simulink model "ControlModel"  (R2020b)
settings: Solver=VariableStepAuto  StartTime=0.0  StopTime=3  FixedStep=0.00001  RelTol=1e-3
InitFcn:
  | s = tf('s');
  | Telec = 1/10000000;
  | Tmech = Telec * 10;
  | CW = 1;
  | CCW = -1;
undefined symbols (not defined in the file or in its folder): DiscIntNeverNeededParam, lag, lead, magnitude, notch, rad
libraries: cstblocks x41, sharedtransform x7, simulink x6, aerolibutil x4, aerolibconvert2 x4, simulink_extras x3, sharedutil x1
(part 2 of 2)

== system ControlModel/Motor + Rotors Model/Current Controller ==
  Current_error : Inport
  Discrete-Time Integrator : DiscreteIntegrator  SampleTime=Telec  ICPrevOutput=DiscIntNeverNeededParam  ICPrevScaledInput=DiscIntNeverNeededParam
  Gain : Gain  Gain=db2mag(65)
  Lag : Subsystem  mask{Beta=10000, Freq=300}
      mask prompts: Beta "Beta ="; Freq "Freq [rad/sec] ="
      mask DialogControl DescTextVar Prompt: Lag controller. Choose the frequency and beta.
      mask Display: disp('Lag')
  Lag1 : Subsystem  Commented=on  mask{Beta=10000, Freq=300}
      mask prompts: Beta "Beta ="; Freq "Freq [rad/sec] ="
      mask DialogControl DescTextVar Prompt: Lag controller. Choose the frequency and beta.
      mask Display: disp('Lag')
  Lead : Subsystem  mask{Phase=60, Freq=2*pi*1000}
      mask prompts: Phase "Phase [deg] ="; Freq "Freq [rad/sec] ="
      mask DialogControl DescTextVar Prompt: First order lead controller. Choose the phase you want and the desired frequency.
      mask Display: disp('Lead')
  Notch : Subsystem  Commented=on  mask{wn=20, wd=20, zn=20, zd=20}
      mask prompts: wn "w_n [rad/sec]"; wd "w_d [rad/sec]"; zn "z_n"; zd "z_d"
      mask DialogControl DescTextVar Prompt: Notch filter
      mask Display: disp('Notch')
  Subsystem1 : Subsystem  Commented=on  mask{Phase=20, Freq=4500}
      mask prompts: Phase "Phase [deg] ="; Freq "Freq [rad/sec] ="
      mask DialogControl DescTextVar Prompt: First order lead controller. Choose the phase you want and the desired frequency.
      mask Display: disp('Lead')
  Voltage_cmd : Outport
  wires:
  Lead/1(Out1) -> Gain/1
  Current_error/1 -> Lag/1(In1)
  Discrete-Time Integrator/1 -> Voltage_cmd/1
  Lag/1(Out1) -> Lead/1(In1)
  Gain/1 -> Discrete-Time Integrator/1

== system ControlModel/Motor + Rotors Model/Plant ==
  V_cmd : Inport
  Gain : Gain  Gain=Kt
  Gain1 : Gain  Gain=Kb
  Scope : Scope  NumInputPorts=2
  Subsystem : Subsystem
      mask Display:
      | disp('1\n')
      | disp('\n----------')
      | disp('\n\n\nLs+R')
  Subsystem1 : Subsystem
      mask Display:
      | disp('1\n')
      | disp('\n----------')
      | disp('\n\n\nJm*s')
  Subsystem2 : Subsystem
      mask Display:
      | disp('1\n')
      | disp('\n----------')
      | disp('\n\n\nJl*s')
  Subsystem3 : Subsystem
  Sum : Sum  Inputs=|+-
  Sum1 : Sum  Inputs=|+-
  Sum2 : Sum  Inputs=-+|
  Im : Outport
  omega : Outport  Port=2
  wires:
  Gain/1 -> Sum2/2
  Sum2/1 -> Subsystem1/1(In1)
  Subsystem3/1(Tload) -> Subsystem2/1(In1), Sum2/1
  Sum1/1 -> Subsystem3/1(dvel)
  Subsystem1/1(Out1) -> Gain1/1, Sum1/1
  Gain1/1 -> Scope/2, Sum/2  "FB"
  V_cmd/1 -> Scope/1, Sum/1  "cmd"
  Sum/1 -> Subsystem/1(In1)
  Subsystem2/1(Out1) -> omega/1, Sum1/2
  Subsystem/1(Im) -> Im/1, Gain/1

== system ControlModel/Motor + Rotors Model/Velocity Controller ==
  Velocity_error : Inport
  Gain : Gain  Gain=db2mag(-42)
  Lag1 : Subsystem  Commented=on  mask{Beta=10000, Freq=300}
      mask prompts: Beta "Beta ="; Freq "Freq [rad/sec] ="
      mask DialogControl DescTextVar Prompt: Lag controller. Choose the frequency and beta.
      mask Display: disp('Lag')
  Notch : Subsystem  Commented=on  mask{wn=20, wd=20, zn=20, zd=20}
      mask prompts: wn "w_n [rad/sec]"; wd "w_d [rad/sec]"; zn "z_n"; zd "z_d"
      mask DialogControl DescTextVar Prompt: Notch filter
      mask Display: disp('Notch')
  Subsystem1 : Subsystem  Commented=on  mask{Phase=20, Freq=4500}
      mask prompts: Phase "Phase [deg] ="; Freq "Freq [rad/sec] ="
      mask DialogControl DescTextVar Prompt: First order lead controller. Choose the phase you want and the desired frequency.
      mask Display: disp('Lead')
  Current_cmd : Outport
  wires:
  Gain/1 -> Current_cmd/1
  Velocity_error/1 -> Gain/1

== system ControlModel/Motor + Rotors Model1/Current Controller ==
  Current_error : Inport
  Discrete-Time Integrator : DiscreteIntegrator  SampleTime=Telec  ICPrevOutput=DiscIntNeverNeededParam  ICPrevScaledInput=DiscIntNeverNeededParam
  Gain : Gain  Gain=db2mag(65)
  Lag : Subsystem  mask{Beta=10000, Freq=300}
      mask prompts: Beta "Beta ="; Freq "Freq [rad/sec] ="
      mask DialogControl DescTextVar Prompt: Lag controller. Choose the frequency and beta.
      mask Display: disp('Lag')
  Lag1 : Subsystem  Commented=on  mask{Beta=10000, Freq=300}
      mask prompts: Beta "Beta ="; Freq "Freq [rad/sec] ="
      mask DialogControl DescTextVar Prompt: Lag controller. Choose the frequency and beta.
      mask Display: disp('Lag')
  Lead : Subsystem  mask{Phase=60, Freq=2*pi*1000}
      mask prompts: Phase "Phase [deg] ="; Freq "Freq [rad/sec] ="
      mask DialogControl DescTextVar Prompt: First order lead controller. Choose the phase you want and the desired frequency.
      mask Display: disp('Lead')
  Notch : Subsystem  Commented=on  mask{wn=20, wd=20, zn=20, zd=20}
      mask prompts: wn "w_n [rad/sec]"; wd "w_d [rad/sec]"; zn "z_n"; zd "z_d"
      mask DialogControl DescTextVar Prompt: Notch filter
      mask Display: disp('Notch')
  Subsystem1 : Subsystem  Commented=on  mask{Phase=20, Freq=4500}
      mask prompts: Phase "Phase [deg] ="; Freq "Freq [rad/sec] ="
      mask DialogControl DescTextVar Prompt: First order lead controller. Choose the phase you want and the desired frequency.
      mask Display: disp('Lead')
  Voltage_cmd : Outport
  wires:
  Lead/1(Out1) -> Gain/1
  Current_error/1 -> Lag/1(In1)
  Discrete-Time Integrator/1 -> Voltage_cmd/1
  Lag/1(Out1) -> Lead/1(In1)
  Gain/1 -> Discrete-Time Integrator/1

== system ControlModel/Motor + Rotors Model1/Subsystem4 ==
  V_cmd : Inport
  Gain : Gain  Gain=Kt
  Gain1 : Gain  Gain=Kb
  Scope : Scope  NumInputPorts=2
  Subsystem : Subsystem
      mask Display:
      | disp('1\n')
      | disp('\n----------')
      | disp('\n\n\nLs+R')
  Subsystem1 : Subsystem
      mask Display:
      | disp('1\n')
      | disp('\n----------')
      | disp('\n\n\nJm*s')
  Subsystem2 : Subsystem
      mask Display:
      | disp('1\n')
      | disp('\n----------')
      | disp('\n\n\nJl*s')
  Subsystem3 : Subsystem
  Sum : Sum  Inputs=|+-
  Sum1 : Sum  Inputs=|+-
  Sum2 : Sum  Inputs=-+|
  Im : Outport
  omega : Outport  Port=2
  wires:
  Gain/1 -> Sum2/2
  Sum2/1 -> Subsystem1/1(In1)
  Subsystem3/1(Tload) -> Subsystem2/1(In1), Sum2/1
  Sum1/1 -> Subsystem3/1(dvel)
  Subsystem1/1(Out1) -> Gain1/1, Sum1/1
  Gain1/1 -> Scope/2, Sum/2  "FB"
  V_cmd/1 -> Scope/1, Sum/1  "cmd"
  Sum/1 -> Subsystem/1(In1)
  Subsystem2/1(Out1) -> omega/1, Sum1/2
  Subsystem/1(Im) -> Im/1, Gain/1

== system ControlModel/Motor + Rotors Model1/Velocity Controller ==
  Velocity_error : Inport
  Gain : Gain  Gain=db2mag(-42)
  Lag1 : Subsystem  Commented=on  mask{Beta=10000, Freq=300}
      mask prompts: Beta "Beta ="; Freq "Freq [rad/sec] ="
      mask DialogControl DescTextVar Prompt: Lag controller. Choose the frequency and beta.
      mask Display: disp('Lag')
  Notch : Subsystem  Commented=on  mask{wn=20, wd=20, zn=20, zd=20}
      mask prompts: wn "w_n [rad/sec]"; wd "w_d [rad/sec]"; zn "z_n"; zd "z_d"
      mask DialogControl DescTextVar Prompt: Notch filter
      mask Display: disp('Notch')
  Subsystem1 : Subsystem  Commented=on  mask{Phase=20, Freq=4500}
      mask prompts: Phase "Phase [deg] ="; Freq "Freq [rad/sec] ="
      mask DialogControl DescTextVar Prompt: First order lead controller. Choose the phase you want and the desired frequency.
      mask Display: disp('Lead')
  Current_cmd : Outport
  wires:
  Gain/1 -> Current_cmd/1
  Velocity_error/1 -> Gain/1

== system ControlModel/Motor + Rotors Model2/Current Controller ==
  Current_error : Inport
  Discrete-Time Integrator : DiscreteIntegrator  SampleTime=Telec  ICPrevOutput=DiscIntNeverNeededParam  ICPrevScaledInput=DiscIntNeverNeededParam
  Gain : Gain  Gain=db2mag(65)
  Lag : Subsystem  mask{Beta=10000, Freq=300}
      mask prompts: Beta "Beta ="; Freq "Freq [rad/sec] ="
      mask DialogControl DescTextVar Prompt: Lag controller. Choose the frequency and beta.
      mask Display: disp('Lag')
  Lag1 : Subsystem  Commented=on  mask{Beta=10000, Freq=300}
      mask prompts: Beta "Beta ="; Freq "Freq [rad/sec] ="
      mask DialogControl DescTextVar Prompt: Lag controller. Choose the frequency and beta.
      mask Display: disp('Lag')
  Lead : Subsystem  mask{Phase=60, Freq=2*pi*1000}
      mask prompts: Phase "Phase [deg] ="; Freq "Freq [rad/sec] ="
      mask DialogControl DescTextVar Prompt: First order lead controller. Choose the phase you want and the desired frequency.
      mask Display: disp('Lead')
  Notch : Subsystem  Commented=on  mask{wn=20, wd=20, zn=20, zd=20}
      mask prompts: wn "w_n [rad/sec]"; wd "w_d [rad/sec]"; zn "z_n"; zd "z_d"
      mask DialogControl DescTextVar Prompt: Notch filter
      mask Display: disp('Notch')
  Subsystem1 : Subsystem  Commented=on  mask{Phase=20, Freq=4500}
      mask prompts: Phase "Phase [deg] ="; Freq "Freq [rad/sec] ="
      mask DialogControl DescTextVar Prompt: First order lead controller. Choose the phase you want and the desired frequency.
      mask Display: disp('Lead')
  Voltage_cmd : Outport
  wires:
  Lead/1(Out1) -> Gain/1
  Current_error/1 -> Lag/1(In1)
  Discrete-Time Integrator/1 -> Voltage_cmd/1
  Lag/1(Out1) -> Lead/1(In1)
  Gain/1 -> Discrete-Time Integrator/1

== system ControlModel/Motor + Rotors Model2/Subsystem4 ==
  V_cmd : Inport
  Gain : Gain  Gain=Kt
  Gain1 : Gain  Gain=Kb
  Scope : Scope  NumInputPorts=2
  Subsystem : Subsystem
      mask Display:
      | disp('1\n')
      | disp('\n----------')
      | disp('\n\n\nLs+R')
  Subsystem1 : Subsystem
      mask Display:
      | disp('1\n')
      | disp('\n----------')
      | disp('\n\n\nJm*s')
  Subsystem2 : Subsystem
      mask Display:
      | disp('1\n')
      | disp('\n----------')
      | disp('\n\n\nJl*s')
  Subsystem3 : Subsystem
  Sum : Sum  Inputs=|+-
  Sum1 : Sum  Inputs=|+-
  Sum2 : Sum  Inputs=-+|
  Im : Outport
  omega : Outport  Port=2
  wires:
  Gain/1 -> Sum2/2
  Sum2/1 -> Subsystem1/1(In1)
  Subsystem3/1(Tload) -> Subsystem2/1(In1), Sum2/1
  Sum1/1 -> Subsystem3/1(dvel)
  Subsystem1/1(Out1) -> Gain1/1, Sum1/1
  Gain1/1 -> Scope/2, Sum/2  "FB"
  V_cmd/1 -> Scope/1, Sum/1  "cmd"
  Sum/1 -> Subsystem/1(In1)
  Subsystem2/1(Out1) -> omega/1, Sum1/2
  Subsystem/1(Im) -> Im/1, Gain/1

== system ControlModel/Motor + Rotors Model2/Velocity Controller ==
  Velocity_error : Inport
  Gain : Gain  Gain=db2mag(-42)
  Lag1 : Subsystem  Commented=on  mask{Beta=10000, Freq=300}
      mask prompts: Beta "Beta ="; Freq "Freq [rad/sec] ="
      mask DialogControl DescTextVar Prompt: Lag controller. Choose the frequency and beta.
      mask Display: disp('Lag')
  Notch : Subsystem  Commented=on  mask{wn=20, wd=20, zn=20, zd=20}
      mask prompts: wn "w_n [rad/sec]"; wd "w_d [rad/sec]"; zn "z_n"; zd "z_d"
      mask DialogControl DescTextVar Prompt: Notch filter
      mask Display: disp('Notch')
  Subsystem1 : Subsystem  Commented=on  mask{Phase=20, Freq=4500}
      mask prompts: Phase "Phase [deg] ="; Freq "Freq [rad/sec] ="
      mask DialogControl DescTextVar Prompt: First order lead controller. Choose the phase you want and the desired frequency.
      mask Display: disp('Lead')
  Current_cmd : Outport
  wires:
  Gain/1 -> Current_cmd/1
  Velocity_error/1 -> Gain/1

== system ControlModel/Motor + Rotors Model3/Current Controller ==
  Current_error : Inport
  Discrete-Time Integrator : DiscreteIntegrator  SampleTime=Telec  ICPrevOutput=DiscIntNeverNeededParam  ICPrevScaledInput=DiscIntNeverNeededParam
  Gain : Gain  Gain=db2mag(65)
  Lag : Subsystem  mask{Beta=10000, Freq=300}
      mask prompts: Beta "Beta ="; Freq "Freq [rad/sec] ="
      mask DialogControl DescTextVar Prompt: Lag controller. Choose the frequency and beta.
      mask Display: disp('Lag')
  Lag1 : Subsystem  Commented=on  mask{Beta=10000, Freq=300}
      mask prompts: Beta "Beta ="; Freq "Freq [rad/sec] ="
      mask DialogControl DescTextVar Prompt: Lag controller. Choose the frequency and beta.
      mask Display: disp('Lag')
  Lead : Subsystem  mask{Phase=60, Freq=2*pi*1000}
      mask prompts: Phase "Phase [deg] ="; Freq "Freq [rad/sec] ="
      mask DialogControl DescTextVar Prompt: First order lead controller. Choose the phase you want and the desired frequency.
      mask Display: disp('Lead')
  Notch : Subsystem  Commented=on  mask{wn=20, wd=20, zn=20, zd=20}
      mask prompts: wn "w_n [rad/sec]"; wd "w_d [rad/sec]"; zn "z_n"; zd "z_d"
      mask DialogControl DescTextVar Prompt: Notch filter
      mask Display: disp('Notch')
  Subsystem1 : Subsystem  Commented=on  mask{Phase=20, Freq=4500}
      mask prompts: Phase "Phase [deg] ="; Freq "Freq [rad/sec] ="
      mask DialogControl DescTextVar Prompt: First order lead controller. Choose the phase you want and the desired frequency.
      mask Display: disp('Lead')
  Voltage_cmd : Outport
  wires:
  Lead/1(Out1) -> Gain/1
  Current_error/1 -> Lag/1(In1)
  Discrete-Time Integrator/1 -> Voltage_cmd/1
  Lag/1(Out1) -> Lead/1(In1)
  Gain/1 -> Discrete-Time Integrator/1

== system ControlModel/Motor + Rotors Model3/Subsystem4 ==
  V_cmd : Inport
  Gain : Gain  Gain=Kt
  Gain1 : Gain  Gain=Kb
  Scope : Scope  NumInputPorts=2
  Subsystem : Subsystem
      mask Display:
      | disp('1\n')
      | disp('\n----------')
      | disp('\n\n\nLs+R')
  Subsystem1 : Subsystem
      mask Display:
      | disp('1\n')
      | disp('\n----------')
      | disp('\n\n\nJm*s')
  Subsystem2 : Subsystem
      mask Display:
      | disp('1\n')
      | disp('\n----------')
      | disp('\n\n\nJl*s')
  Subsystem3 : Subsystem
  Sum : Sum  Inputs=|+-
  Sum1 : Sum  Inputs=|+-
  Sum2 : Sum  Inputs=-+|
  Im : Outport
  omega : Outport  Port=2
  wires:
  Gain/1 -> Sum2/2
  Sum2/1 -> Subsystem1/1(In1)
  Subsystem3/1(Tload) -> Subsystem2/1(In1), Sum2/1
  Sum1/1 -> Subsystem3/1(dvel)
  Subsystem1/1(Out1) -> Gain1/1, Sum1/1
  Gain1/1 -> Scope/2, Sum/2  "FB"
  V_cmd/1 -> Scope/1, Sum/1  "cmd"
  Sum/1 -> Subsystem/1(In1)
  Subsystem2/1(Out1) -> omega/1, Sum1/2
  Subsystem/1(Im) -> Im/1, Gain/1

== system ControlModel/Motor + Rotors Model3/Velocity Controller ==
  Velocity_error : Inport
  Gain : Gain  Gain=db2mag(-42)
  Lag1 : Subsystem  Commented=on  mask{Beta=10000, Freq=300}
      mask prompts: Beta "Beta ="; Freq "Freq [rad/sec] ="
      mask DialogControl DescTextVar Prompt: Lag controller. Choose the frequency and beta.
      mask Display: disp('Lag')
  Notch : Subsystem  Commented=on  mask{wn=20, wd=20, zn=20, zd=20}
      mask prompts: wn "w_n [rad/sec]"; wd "w_d [rad/sec]"; zn "z_n"; zd "z_d"
      mask DialogControl DescTextVar Prompt: Notch filter
      mask Display: disp('Notch')
  Subsystem1 : Subsystem  Commented=on  mask{Phase=20, Freq=4500}
      mask prompts: Phase "Phase [deg] ="; Freq "Freq [rad/sec] ="
      mask DialogControl DescTextVar Prompt: First order lead controller. Choose the phase you want and the desired frequency.
      mask Display: disp('Lead')
  Current_cmd : Outport
  wires:
  Gain/1 -> Current_cmd/1
  Velocity_error/1 -> Gain/1

== system ControlModel/Attitude Controller/Old Calculations/Quaternions Transformation ==
  acc : Inport
  Yaw.SP : Inport  Port=2
  phi,theta,psi : Inport  Port=3
  Acceleration to quaternion : MATLAB Function  TreatAsAtomicUnit=on
  Add : Sum  Inputs=+-
  Product : Product
  Quaternion Norm : sharedutil/Quaternion Norm  aMode=aMode
      settings: SourceProductBaseCode=AE,PW,MT,UV,VE,VP
  Quaternions to Rotation Angles : sharedtransform/Quaternions to Rotation Angles  rotationOrder=ZYX  aMode=aMode
      settings: SourceProductBaseCode=AE,PW,MT,UV,VE,VP
  Rotation Angles to Quaternions : sharedtransform/Rotation Angles to Quaternions  rotationOrder=ZYX  aMode=aMode
      settings: SourceProductBaseCode=AE,PW,MT,UV,VE,VP
  Sign : Signum
  Out1 : Outport
  wires:
  phi,theta,psi/1 -> Rotation Angles to Quaternions/1, Acceleration to quaternion/2(angles)
  Add/1 -> Quaternions to Rotation Angles/1, Quaternion Norm/1
  Quaternions to Rotation Angles/1 -> Product/2
  Rotation Angles to Quaternions/1 -> Add/2, Acceleration to quaternion/3(q)
  acc/1 -> Acceleration to quaternion/1(acc)
  Sign/1 -> Product/1
  Quaternion Norm/1 -> Sign/1
  Yaw.SP/1 -> Acceleration to quaternion/4(psi_sp)
  Acceleration to quaternion/1(qcmd) -> Add/1
  Product/1 -> Out1/1

== system ControlModel/Attitude Controller/Old Calculations/Quaternions Transformation - New Version ==
  acc : Inport
  Yaw.SP : Inport  Port=2
  phi,theta,psi : Inport  Port=3
  Acceleration 2 quaternion - continue : MATLAB Function  TreatAsAtomicUnit=on
  Acceleration to quaternion - new Version : MATLAB Function  TreatAsAtomicUnit=on
  Quaternion Inverse : aerolibutil/Quaternion Inverse
  Quaternion Multiplication : aerolibutil/Quaternion Multiplication
  Quaternion Multiplication1 : aerolibutil/Quaternion Multiplication
  Quaternion Rotation : aerolibutil/Quaternion Rotation
  Rotation Angles to Quaternions : sharedtransform/Rotation Angles to Quaternions  rotationOrder=ZYX  aMode=aMode
      settings: SourceProductBaseCode=AE,PW,MT,UV,VE,VP
  Rotation Angles to Quaternions1 : sharedtransform/Rotation Angles to Quaternions  rotationOrder=ZYX  aMode=aMode
      settings: SourceProductBaseCode=AE,PW,MT,UV,VE,VP
  signDecision : MATLAB Function  TreatAsAtomicUnit=on
  q_e_rp : Outport
  q_e_y : Outport  Port=2
  wires:
  acc/1 -> Acceleration to quaternion - new Version/3(acc)
  phi,theta,psi/1 -> Acceleration to quaternion - new Version/2(angles), Rotation Angles to Quaternions/1
  Rotation Angles to Quaternions/1 -> Acceleration to quaternion - new Version/1("q ")
  Acceleration to quaternion - new Version/4(Ieb_cmd_z) -> Acceleration 2 quaternion - continue/4(Ieb_cmd_z)
  Acceleration to quaternion - new Version/3(alpha) -> Acceleration 2 quaternion - continue/3(alpha)
  Yaw.SP/1 -> Acceleration 2 quaternion - continue/5(psi_sp)
  Acceleration to quaternion - new Version/1(q) -> Acceleration 2 quaternion - continue/1(q), Quaternion Multiplication1/1, Quaternion Rotation/1
  Acceleration to quaternion - new Version/2(N) -> Quaternion Rotation/2
  Quaternion Rotation/1 -> Acceleration 2 quaternion - continue/2(Nb)
  Acceleration 2 quaternion - continue/1(qerp_not_quat) -> Quaternion Multiplication1/2, signDecision/1(u)
  Acceleration 2 quaternion - continue/2(eul) -> Rotation Angles to Quaternions1/1
  Rotation Angles to Quaternions1/1 -> Quaternion Multiplication/1  "qdes"
  Quaternion Inverse/1 -> Quaternion Multiplication/2
  Quaternion Multiplication1/1 -> Quaternion Inverse/1
  Quaternion Multiplication/1 -> q_e_y/1
  signDecision/1(y) -> q_e_rp/1

== system ControlModel/Motor + Rotors Model/Current Controller/Lag ==
  In1 : Inport
  LTI System : cstblocks/LTI System  sys=c2d(lag(Freq,Beta),Telec)  IC=[]
  Out1 : Outport
  wires:
  LTI System/1 -> Out1/1
  In1/1 -> LTI System/1

== system ControlModel/Motor + Rotors Model/Current Controller/Lag1 ==
  In1 : Inport
  LTI System : cstblocks/LTI System  sys=lag(Freq,Beta)  IC=[]
  Out1 : Outport
  wires:
  In1/1 -> LTI System/1
  LTI System/1 -> Out1/1

== system ControlModel/Motor + Rotors Model/Current Controller/Lead ==
  In1 : Inport
  LTI System : cstblocks/LTI System  sys=c2d(lead(Phase,Freq),Telec)  IC=[]
  Out1 : Outport
  wires:
  LTI System/1 -> Out1/1
  In1/1 -> LTI System/1

== system ControlModel/Motor + Rotors Model/Current Controller/Notch ==
  In1 : Inport
  LTI System : cstblocks/LTI System  sys=notch(wn,wd,zn,zd)  IC=[]
  Out1 : Outport
  wires:
  LTI System/1 -> Out1/1
  In1/1 -> LTI System/1

== system ControlModel/Motor + Rotors Model/Current Controller/Subsystem1 ==
  In1 : Inport
  LTI System : cstblocks/LTI System  sys=lead(Phase,Freq)  IC=[]
  Out1 : Outport
  wires:
  In1/1 -> LTI System/1
  LTI System/1 -> Out1/1

== system ControlModel/Motor + Rotors Model/Plant/Subsystem ==
  In1 : Inport
  Discrete-Time Integrator : DiscreteIntegrator  SampleTime=-1  ICPrevOutput=DiscIntNeverNeededParam  ICPrevScaledInput=DiscIntNeverNeededParam
  Gain : Gain  Gain=R
  Gain1 : Gain  Gain=1/L
  Sum : Sum  Inputs=|+-
  Im : Outport
  wires:
  Gain/1 -> Sum/2
  Gain1/1 -> Discrete-Time Integrator/1
  Discrete-Time Integrator/1 -> Im/1, Gain/1
  Sum/1 -> Gain1/1
  In1/1 -> Sum/1

== system ControlModel/Motor + Rotors Model/Plant/Subsystem1 ==
  In1 : Inport
  Discrete-Time Integrator : DiscreteIntegrator  SampleTime=Telec  ICPrevOutput=DiscIntNeverNeededParam  ICPrevScaledInput=DiscIntNeverNeededParam
  Gain : Gain  Gain=1/Jm
  Out1 : Outport
  wires:
  Gain/1 -> Out1/1
  Discrete-Time Integrator/1 -> Gain/1
  In1/1 -> Discrete-Time Integrator/1

== system ControlModel/Motor + Rotors Model/Plant/Subsystem2 ==
  In1 : Inport
  Discrete-Time Integrator : DiscreteIntegrator  SampleTime=Telec  ICPrevOutput=DiscIntNeverNeededParam  ICPrevScaledInput=DiscIntNeverNeededParam
  Gain : Gain  Gain=1/Jl
  Out1 : Outport
  wires:
  Gain/1 -> Out1/1
  In1/1 -> Discrete-Time Integrator/1
  Discrete-Time Integrator/1 -> Gain/1

== system ControlModel/Motor + Rotors Model/Plant/Subsystem3 ==
  dvel : Inport
  Add : Sum
  Discrete-Time Integrator : DiscreteIntegrator  SampleTime=Telec  ICPrevOutput=DiscIntNeverNeededParam  ICPrevScaledInput=DiscIntNeverNeededParam
  Gain2 : Gain  Gain=Kv
  Gain5 : Gain  Gain=Kk
  Tload : Outport
  wires:
  Add/1 -> Tload/1
  Gain2/1 -> Add/1
  Gain5/1 -> Add/2
  dvel/1 -> Discrete-Time Integrator/1, Gain2/1
  Discrete-Time Integrator/1 -> Gain5/1

== system ControlModel/Motor + Rotors Model/Velocity Controller/Lag1 ==
  In1 : Inport
  LTI System : cstblocks/LTI System  sys=lag(Freq,Beta)  IC=[]
  Out1 : Outport
  wires:
  In1/1 -> LTI System/1
  LTI System/1 -> Out1/1

== system ControlModel/Motor + Rotors Model/Velocity Controller/Notch ==
  In1 : Inport
  LTI System : cstblocks/LTI System  sys=notch(wn,wd,zn,zd)  IC=[]
  Out1 : Outport
  wires:
  LTI System/1 -> Out1/1
  In1/1 -> LTI System/1

== system ControlModel/Motor + Rotors Model/Velocity Controller/Subsystem1 ==
  In1 : Inport
  LTI System : cstblocks/LTI System  sys=lead(Phase,Freq)  IC=[]
  Out1 : Outport
  wires:
  In1/1 -> LTI System/1
  LTI System/1 -> Out1/1

== system ControlModel/Motor + Rotors Model1/Current Controller/Lag ==
  In1 : Inport
  LTI System : cstblocks/LTI System  sys=c2d(lag(Freq,Beta),Telec)  IC=[]
  Out1 : Outport
  wires:
  LTI System/1 -> Out1/1
  In1/1 -> LTI System/1

== system ControlModel/Motor + Rotors Model1/Current Controller/Lag1 ==
  In1 : Inport
  LTI System : cstblocks/LTI System  sys=lag(Freq,Beta)  IC=[]
  Out1 : Outport
  wires:
  In1/1 -> LTI System/1
  LTI System/1 -> Out1/1

== system ControlModel/Motor + Rotors Model1/Current Controller/Lead ==
  In1 : Inport
  LTI System : cstblocks/LTI System  sys=c2d(lead(Phase,Freq),Telec)  IC=[]
  Out1 : Outport
  wires:
  LTI System/1 -> Out1/1
  In1/1 -> LTI System/1

== system ControlModel/Motor + Rotors Model1/Current Controller/Notch ==
  In1 : Inport
  LTI System : cstblocks/LTI System  sys=notch(wn,wd,zn,zd)  IC=[]
  Out1 : Outport
  wires:
  LTI System/1 -> Out1/1
  In1/1 -> LTI System/1

== system ControlModel/Motor + Rotors Model1/Current Controller/Subsystem1 ==
  In1 : Inport
  LTI System : cstblocks/LTI System  sys=lead(Phase,Freq)  IC=[]
  Out1 : Outport
  wires:
  In1/1 -> LTI System/1
  LTI System/1 -> Out1/1

== system ControlModel/Motor + Rotors Model1/Subsystem4/Subsystem ==
  In1 : Inport
  Discrete-Time Integrator : DiscreteIntegrator  SampleTime=Telec  ICPrevOutput=DiscIntNeverNeededParam  ICPrevScaledInput=DiscIntNeverNeededParam
  Gain : Gain  Gain=R
  Gain1 : Gain  Gain=1/L
  Sum : Sum  Inputs=|+-
  Im : Outport
  wires:
  Gain/1 -> Sum/2
  Gain1/1 -> Discrete-Time Integrator/1
  Discrete-Time Integrator/1 -> Im/1, Gain/1
  Sum/1 -> Gain1/1
  In1/1 -> Sum/1

== system ControlModel/Motor + Rotors Model1/Subsystem4/Subsystem1 ==
  In1 : Inport
  Discrete-Time Integrator : DiscreteIntegrator  SampleTime=Telec  ICPrevOutput=DiscIntNeverNeededParam  ICPrevScaledInput=DiscIntNeverNeededParam
  Gain : Gain  Gain=1/Jm
  Out1 : Outport
  wires:
  Gain/1 -> Out1/1
  Discrete-Time Integrator/1 -> Gain/1
  In1/1 -> Discrete-Time Integrator/1

== system ControlModel/Motor + Rotors Model1/Subsystem4/Subsystem2 ==
  In1 : Inport
  Discrete-Time Integrator : DiscreteIntegrator  SampleTime=Telec  ICPrevOutput=DiscIntNeverNeededParam  ICPrevScaledInput=DiscIntNeverNeededParam
  Gain : Gain  Gain=1/Jl
  Out1 : Outport
  wires:
  Gain/1 -> Out1/1
  In1/1 -> Discrete-Time Integrator/1
  Discrete-Time Integrator/1 -> Gain/1

== system ControlModel/Motor + Rotors Model1/Subsystem4/Subsystem3 ==
  dvel : Inport
  Add : Sum
  Discrete-Time Integrator : DiscreteIntegrator  SampleTime=Telec  ICPrevOutput=DiscIntNeverNeededParam  ICPrevScaledInput=DiscIntNeverNeededParam
  Gain2 : Gain  Gain=Kv
  Gain5 : Gain  Gain=Kk
  Tload : Outport
  wires:
  Add/1 -> Tload/1
  Gain2/1 -> Add/1
  Gain5/1 -> Add/2
  dvel/1 -> Discrete-Time Integrator/1, Gain2/1
  Discrete-Time Integrator/1 -> Gain5/1

== system ControlModel/Motor + Rotors Model1/Velocity Controller/Lag1 ==
  In1 : Inport
  LTI System : cstblocks/LTI System  sys=lag(Freq,Beta)  IC=[]
  Out1 : Outport
  wires:
  LTI System/1 -> Out1/1
  In1/1 -> LTI System/1

== system ControlModel/Motor + Rotors Model1/Velocity Controller/Notch ==
  In1 : Inport
  LTI System : cstblocks/LTI System  sys=notch(wn,wd,zn,zd)  IC=[]
  Out1 : Outport
  wires:
  In1/1 -> LTI System/1
  LTI System/1 -> Out1/1

== system ControlModel/Motor + Rotors Model1/Velocity Controller/Subsystem1 ==
  In1 : Inport
  LTI System : cstblocks/LTI System  sys=lead(Phase,Freq)  IC=[]
  Out1 : Outport
  wires:
  LTI System/1 -> Out1/1
  In1/1 -> LTI System/1

== system ControlModel/Motor + Rotors Model2/Current Controller/Lag ==
  In1 : Inport
  LTI System : cstblocks/LTI System  sys=c2d(lag(Freq,Beta),Telec)  IC=[]
  Out1 : Outport
  wires:
  LTI System/1 -> Out1/1
  In1/1 -> LTI System/1

== system ControlModel/Motor + Rotors Model2/Current Controller/Lag1 ==
  In1 : Inport
  LTI System : cstblocks/LTI System  sys=lag(Freq,Beta)  IC=[]
  Out1 : Outport
  wires:
  In1/1 -> LTI System/1
  LTI System/1 -> Out1/1

== system ControlModel/Motor + Rotors Model2/Current Controller/Lead ==
  In1 : Inport
  LTI System : cstblocks/LTI System  sys=c2d(lead(Phase,Freq),Telec)  IC=[]
  Out1 : Outport
  wires:
  LTI System/1 -> Out1/1
  In1/1 -> LTI System/1

== system ControlModel/Motor + Rotors Model2/Current Controller/Notch ==
  In1 : Inport
  LTI System : cstblocks/LTI System  sys=notch(wn,wd,zn,zd)  IC=[]
  Out1 : Outport
  wires:
  LTI System/1 -> Out1/1
  In1/1 -> LTI System/1

== system ControlModel/Motor + Rotors Model2/Current Controller/Subsystem1 ==
  In1 : Inport
  LTI System : cstblocks/LTI System  sys=lead(Phase,Freq)  IC=[]
  Out1 : Outport
  wires:
  In1/1 -> LTI System/1
  LTI System/1 -> Out1/1

== system ControlModel/Motor + Rotors Model2/Subsystem4/Subsystem ==
  In1 : Inport
  Discrete-Time Integrator : DiscreteIntegrator  SampleTime=Telec  ICPrevOutput=DiscIntNeverNeededParam  ICPrevScaledInput=DiscIntNeverNeededParam
  Gain : Gain  Gain=R
  Gain1 : Gain  Gain=1/L
  Sum : Sum  Inputs=|+-
  Im : Outport
  wires:
  Gain/1 -> Sum/2
  Gain1/1 -> Discrete-Time Integrator/1
  Discrete-Time Integrator/1 -> Im/1, Gain/1
  Sum/1 -> Gain1/1
  In1/1 -> Sum/1

== system ControlModel/Motor + Rotors Model2/Subsystem4/Subsystem1 ==
  In1 : Inport
  Discrete-Time Integrator : DiscreteIntegrator  SampleTime=Telec  ICPrevOutput=DiscIntNeverNeededParam  ICPrevScaledInput=DiscIntNeverNeededParam
  Gain : Gain  Gain=1/Jm
  Out1 : Outport
  wires:
  Gain/1 -> Out1/1
  Discrete-Time Integrator/1 -> Gain/1
  In1/1 -> Discrete-Time Integrator/1

== system ControlModel/Motor + Rotors Model2/Subsystem4/Subsystem2 ==
  In1 : Inport
  Discrete-Time Integrator : DiscreteIntegrator  SampleTime=Telec  ICPrevOutput=DiscIntNeverNeededParam  ICPrevScaledInput=DiscIntNeverNeededParam
  Gain : Gain  Gain=1/Jl
  Out1 : Outport
  wires:
  Gain/1 -> Out1/1
  In1/1 -> Discrete-Time Integrator/1
  Discrete-Time Integrator/1 -> Gain/1

== system ControlModel/Motor + Rotors Model2/Subsystem4/Subsystem3 ==
  dvel : Inport
  Add : Sum
  Discrete-Time Integrator : DiscreteIntegrator  SampleTime=Telec  ICPrevOutput=DiscIntNeverNeededParam  ICPrevScaledInput=DiscIntNeverNeededParam
  Gain2 : Gain  Gain=Kv
  Gain5 : Gain  Gain=Kk
  Tload : Outport
  wires:
  Add/1 -> Tload/1
  Gain2/1 -> Add/1
  Gain5/1 -> Add/2
  dvel/1 -> Discrete-Time Integrator/1, Gain2/1
  Discrete-Time Integrator/1 -> Gain5/1

== system ControlModel/Motor + Rotors Model2/Velocity Controller/Lag1 ==
  In1 : Inport
  LTI System : cstblocks/LTI System  sys=lag(Freq,Beta)  IC=[]
  Out1 : Outport
  wires:
  In1/1 -> LTI System/1
  LTI System/1 -> Out1/1

== system ControlModel/Motor + Rotors Model2/Velocity Controller/Notch ==
  In1 : Inport
  LTI System : cstblocks/LTI System  sys=notch(wn,wd,zn,zd)  IC=[]
  Out1 : Outport
  wires:
  LTI System/1 -> Out1/1
  In1/1 -> LTI System/1

== system ControlModel/Motor + Rotors Model2/Velocity Controller/Subsystem1 ==
  In1 : Inport
  LTI System : cstblocks/LTI System  sys=lead(Phase,Freq)  IC=[]
  Out1 : Outport
  wires:
  In1/1 -> LTI System/1
  LTI System/1 -> Out1/1

== system ControlModel/Motor + Rotors Model3/Current Controller/Lag ==
  In1 : Inport
  LTI System : cstblocks/LTI System  sys=c2d(lag(Freq,Beta),Telec)  IC=[]
  Out1 : Outport
  wires:
  LTI System/1 -> Out1/1
  In1/1 -> LTI System/1

== system ControlModel/Motor + Rotors Model3/Current Controller/Lag1 ==
  In1 : Inport
  LTI System : cstblocks/LTI System  sys=lag(Freq,Beta)  IC=[]
  Out1 : Outport
  wires:
  In1/1 -> LTI System/1
  LTI System/1 -> Out1/1

== system ControlModel/Motor + Rotors Model3/Current Controller/Lead ==
  In1 : Inport
  LTI System : cstblocks/LTI System  sys=c2d(lead(Phase,Freq),Telec)  IC=[]
  Out1 : Outport
  wires:
  LTI System/1 -> Out1/1
  In1/1 -> LTI System/1

== system ControlModel/Motor + Rotors Model3/Current Controller/Notch ==
  In1 : Inport
  LTI System : cstblocks/LTI System  sys=notch(wn,wd,zn,zd)  IC=[]
  Out1 : Outport
  wires:
  LTI System/1 -> Out1/1
  In1/1 -> LTI System/1

== system ControlModel/Motor + Rotors Model3/Current Controller/Subsystem1 ==
  In1 : Inport
  LTI System : cstblocks/LTI System  sys=lead(Phase,Freq)  IC=[]
  Out1 : Outport
  wires:
  In1/1 -> LTI System/1
  LTI System/1 -> Out1/1

== system ControlModel/Motor + Rotors Model3/Subsystem4/Subsystem ==
  In1 : Inport
  Discrete-Time Integrator : DiscreteIntegrator  SampleTime=Telec  ICPrevOutput=DiscIntNeverNeededParam  ICPrevScaledInput=DiscIntNeverNeededParam
  Gain : Gain  Gain=R
  Gain1 : Gain  Gain=1/L
  Sum : Sum  Inputs=|+-
  Im : Outport
  wires:
  Gain/1 -> Sum/2
  Gain1/1 -> Discrete-Time Integrator/1
  Discrete-Time Integrator/1 -> Im/1, Gain/1
  Sum/1 -> Gain1/1
  In1/1 -> Sum/1

== system ControlModel/Motor + Rotors Model3/Subsystem4/Subsystem1 ==
  In1 : Inport
  Discrete-Time Integrator : DiscreteIntegrator  SampleTime=Telec  ICPrevOutput=DiscIntNeverNeededParam  ICPrevScaledInput=DiscIntNeverNeededParam
  Gain : Gain  Gain=1/Jm
  Out1 : Outport
  wires:
  Gain/1 -> Out1/1
  Discrete-Time Integrator/1 -> Gain/1
  In1/1 -> Discrete-Time Integrator/1

== system ControlModel/Motor + Rotors Model3/Subsystem4/Subsystem2 ==
  In1 : Inport
  Discrete-Time Integrator : DiscreteIntegrator  SampleTime=Telec  ICPrevOutput=DiscIntNeverNeededParam  ICPrevScaledInput=DiscIntNeverNeededParam
  Gain : Gain  Gain=1/Jl
  Out1 : Outport
  wires:
  Gain/1 -> Out1/1
  In1/1 -> Discrete-Time Integrator/1
  Discrete-Time Integrator/1 -> Gain/1

== system ControlModel/Motor + Rotors Model3/Subsystem4/Subsystem3 ==
  dvel : Inport
  Add : Sum
  Discrete-Time Integrator : DiscreteIntegrator  SampleTime=Telec  ICPrevOutput=DiscIntNeverNeededParam  ICPrevScaledInput=DiscIntNeverNeededParam
  Gain2 : Gain  Gain=Kv
  Gain5 : Gain  Gain=Kk
  Tload : Outport
  wires:
  Add/1 -> Tload/1
  Gain2/1 -> Add/1
  Gain5/1 -> Add/2
  dvel/1 -> Discrete-Time Integrator/1, Gain2/1
  Discrete-Time Integrator/1 -> Gain5/1

== system ControlModel/Motor + Rotors Model3/Velocity Controller/Lag1 ==
  In1 : Inport
  LTI System : cstblocks/LTI System  sys=lag(Freq,Beta)  IC=[]
  Out1 : Outport
  wires:
  LTI System/1 -> Out1/1
  In1/1 -> LTI System/1

== system ControlModel/Motor + Rotors Model3/Velocity Controller/Notch ==
  In1 : Inport
  LTI System : cstblocks/LTI System  sys=notch(wn,wd,zn,zd)  IC=[]
  Out1 : Outport
  wires:
  In1/1 -> LTI System/1
  LTI System/1 -> Out1/1

== system ControlModel/Motor + Rotors Model3/Velocity Controller/Subsystem1 ==
  In1 : Inport
  LTI System : cstblocks/LTI System  sys=lead(Phase,Freq)  IC=[]
  Out1 : Outport
  wires:
  LTI System/1 -> Out1/1
  In1/1 -> LTI System/1

== matlab function ControlModel/Attitude Controller/Old Calculations/Euler Angles Transformation ==
  data: acc_ned input; acc_body output; angles input
function acc_body = fcn(acc_ned,angles)
phi = angles(1);
theta = angles(2);
psi = angles(3);
Rotation_Mat = Rot_E2B(theta,psi,phi);

acc_body = Rotation_Mat\acc_ned;

== matlab function ControlModel/Attitude Controller/Old Calculations/Quaternions Transformation/Acceleration to quaternion ==
  data: acc input; qcmd output; angles input; q input; psi_sp input
function qcmd = fcn(acc,angles , q, psi_sp)

% this function transform the acceleration command to quaternion, based on
% the acceleration command, euler angles and the current quaternion
% transformation based on the paper:"Nonlinear Quadrotor Attitude Control,
% Technical Report".
% Iftach Naftaly, 2020.


% getting the rotation matrix from I to B
phi = angles(1);
theta = angles(2);
psi = angles(3);
Rot_ZYX = Rot_E2B(theta,psi,phi);


% dont calculate if the acceleration is 0
if norm(acc) == 0
    acc = [0.1;0.1;0.1];
end

% reduce order quaternion calculation
Ieb_cmd_z = acc/norm(acc);
Ieb_z = Rot_ZYX\[0;0;1];


alpha = acos(Ieb_z.'*Ieb_cmd_z);
CP = cross(Ieb_z,Ieb_cmd_z);
q1_3 = sin(alpha)*CP/norm(CP);
q0 = cos(alpha);
qred = quaternion(q0,q1_3(1),q1_3(2),q1_3(3));
% qcmd_red = q*qred;
qcmd_red = quaternion(0,1,3,1);
%full order quaternion calculation.
cpsi = cos(psi_sp);
spsi = sin(psi_sp);
R_KI = [cpsi spsi 0; -spsi cpsi 0; 0 0 1];
Keb_cmd_z = R_KI*Ieb_cmd_z;

theta_cmd = atan(Keb_cmd_z(1)/Keb_cmd_z(3));
ct = cos(theta_cmd);
st = sin(theta_cmd);
R_LK = [ct 0 -st; 0 1 0; st 0 ct];

Leb_cmd_z = R_LK*Keb_cmd_z;

phi_cmd = atan2(-Leb_cmd_z(2),Leb_cmd_z(3));
qcmd_full = eul2quat([phi_cmd theta_cmd psi_sp]);
% mixing full and reduced attitue control
% qcmd = qcmd_red * quatinv([qcmd_red]) * qcmd_full;
qcmd =qcmd_full;

== matlab function ControlModel/Attitude Controller/MATLAB Function ==
  data: u input; R1 output; R2 output; R3 output
function [R1,R2,R3] = fcn(u)
rot_mat = Rot_E2B(u(1),u(2),u(3));
R1 = rot_mat(:,1);
R2 = rot_mat(:,2);
R3 = rot_mat(:,3);

== matlab function ControlModel/Attitude Controller/Old Calculations/Quaternions Transformation - New Version/Acceleration to quaternion - new Version ==
  data: q output; q input; angles input; acc input; N output; alpha output; Ieb_cmd_z output
function [q, N, alpha, Ieb_cmd_z] = fcn(q, angles, acc)

% this function transform the acceleration command to quaternion, based on
% the acceleration command, euler angles and the current quaternion
% transformation based on the paper:"Quadrotor control for accurate agile flight
%Fässler, Matthias"
% Iftach Naftaly, 2020.


% getting the rotation matrix from I to B
phi = angles(1);
theta = angles(2);
psi = angles(3);
Rot_ZYX = Rot_E2B(theta,psi,phi);
% q = q.';
% dont calculate if the acceleration is 0
if norm(acc) == 0
    acc = [0.01;0.01;0.01];
end

% X-Y plane - Roll and Pitch
Ieb_cmd_z = acc/norm(acc);
Ieb_z = Rot_ZYX\[0;0;1];
alpha = acos(Ieb_z.'*Ieb_cmd_z);
N = cross(Ieb_z,Ieb_cmd_z);

== matlab function ControlModel/Attitude Controller/Old Calculations/Quaternions Transformation - New Version/signDecision ==
  data: u input; y output
function y = fcn(u)

if u(1) > 0
    y = u;
else
    y = -u;
end

== matlab function ControlModel/Attitude Controller/Old Calculations/Quaternions Transformation - New Version/Acceleration 2 quaternion - continue ==
  data: q input; Nb input; alpha input; qerp_not_quat output; Ieb_cmd_z input; psi_sp input; eul output
function [qerp_not_quat,eul] = fcn(q,Nb, alpha, Ieb_cmd_z, psi_sp)

% this function transform the acceleration command to quaternion, based on
% the acceleration command, euler angles and the current quaternion
% transformation based on the paper:"Quadrotor control for accurate agile flight
%Fässler, Matthias" additional code
% Iftach Naftaly, 2020.


%  X - Y Plane
q1_3 = sin(alpha)*Nb/norm(Nb);
q0 = cos(alpha);
qerp = quaternion(q0,q1_3(1),q1_3(2),q1_3(3));
qerp_not_quat = [q0;q1_3];

% Z plane - Yaw
ex_c = [cos(psi_sp);sin(psi_sp);0];
ey_c = [-sin(psi_sp);cos(psi_sp);0];

ex_b_des = cross(ey_c,Ieb_cmd_z)/norm(cross(ey_c,Ieb_cmd_z));
ey_b_des = cross(Ieb_cmd_z,ex_c)/norm(cross(Ieb_cmd_z,ex_c));
Rd = [ex_b_des ey_b_des Ieb_cmd_z];
eul = rotm2eul(Rd);
% 
% qdes = quaternion(ex_b_des,ex_b_des,ey_b_des,Ieb_cmd_z);
% 
% qey = quatmultiply(quatinv(quatmultiply(q,qerp)),qdes);
% qey_not_quad = [qey(1);qey(2);qey(3);qey(4)];

== matlab function ControlModel/Mixer/MATLAB Function ==
  data: mat input; y output; vect input
function y = fcn(mat,vect)
y = mat\vect;

== matlab function ControlModel/Attitude Controller/Acceleration to Quaternions1/quatVect ==
  data: acc input; eulAngles output; des_yaw input; thrust output
function [eulAngles, thrust] = fcn(acc,des_yaw)
%this function calculates the quaternion based on acceleration command and
%desired yaw angle. based on
%https://github.com/Jaeyoung-Lim/mavros_controllers/blob/master/geometric_controller/src/geometric_controller.cpp,
% because of code generation limitations, the output is the rotation
% matrix, then it needs to be converter to quaternions with rot2quat block.
%Iftach Naftaly, 12.2020

proj_xb_des = [cosd(des_yaw);sind(des_yaw);0];

zb_des = acc/norm(acc);
yb_des = cross(zb_des,proj_xb_des)/norm(cross(zb_des,proj_xb_des));
xb_des = cross(yb_des,zb_des)/norm(cross(yb_des,zb_des));


rotMat = [xb_des yb_des zb_des];

eulAngles = rotm2eul(rotMat);

thrust = norm(acc);
